simulink model "caso_scalare_stabilita"  (R2024b)
settings: Solver=VariableStepAuto  StartTime=0.0  StopTime=10.0  RelTol=1e-3
settings Model: Creator=david  LastModifiedBy=david

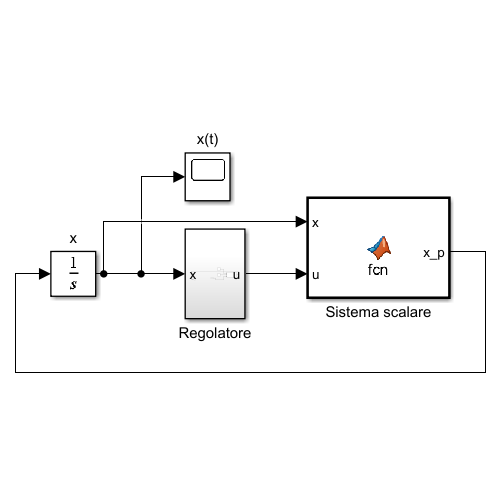
[thumbnail: Simulink's stored preview of the top-level diagram]
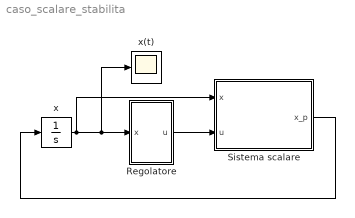
== system caso_scalare_stabilita ==
  Regolatore : Subsystem
  Sistema scalare : MATLAB Function  TreatAsAtomicUnit=on
  x : Integrator  InitialCondition=1
  x(t) : Scope
  wires:
  Sistema scalare/1(x_p) -> x/1
  x/1 -> x(t)/1, Regolatore/1(x), Sistema scalare/1(x)
  Regolatore/1(u) -> Sistema scalare/2(u)

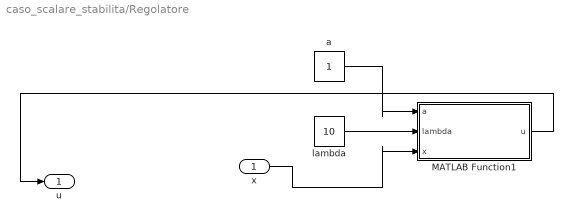
== system caso_scalare_stabilita/Regolatore ==
  x : Inport
  MATLAB Function1 : MATLAB Function  TreatAsAtomicUnit=on
  a : Constant  VectorParams1D=off
  lambda : Constant  Value=10  VectorParams1D=off
  u : Outport
  wires:
  a/1 -> MATLAB Function1/1(a)
  lambda/1 -> MATLAB Function1/2(lambda)
  MATLAB Function1/1(u) -> u/1
  x/1 -> MATLAB Function1/3(x)

== matlab function caso_scalare_stabilita/Sistema scalare ==
  data: x input; x_p output; u input
function x_p = fcn(x,u)


a = 1; %parametro del sistema 
x_p = a*x+u; %evoluzione del sistema

== matlab function caso_scalare_stabilita/Regolatore/MATLAB Function1 ==
  data: a input; lambda input; x input; u output
function u = fcn(a,lambda,x)

k = -a-lambda;
u = k*x; %regolazione
